simulink model "Lidar_Final_Model"  (R2022b)
settings: Solver=VariableStepAuto  StartTime=0.0  StopTime=inf  RelTol=1e-3
model workspace (MAT data in the model file):
  SL_ROS_VariableLengthArrays_MaxSizes.CommonInfo.ArrayTruncateAction = 'EmitWarning'
  SL_ROS_VariableLengthArrays_MaxSizes.MsgTypeMap = containers.Map
  SL_ROS_VariableLengthArrays_MaxSizes.MsgTypeMap.serialization.keys = {'sensor_msgs/PointCloud2', 'sensor_msgs/PointField', 'std_msgs/Header'}
  SL_ROS_VariableLengthArrays_MaxSizes.MsgTypeMap.serialization.values{1}(1).PropertyName = 'Data'
  SL_ROS_VariableLengthArrays_MaxSizes.MsgTypeMap.serialization.values{1}(1).DataType = 'uint8'
  SL_ROS_VariableLengthArrays_MaxSizes.MsgTypeMap.serialization.values{1}(1).MaxLength = 1000000
  SL_ROS_VariableLengthArrays_MaxSizes.MsgTypeMap.serialization.values{1}(2).PropertyName = 'Fields'
  SL_ROS_VariableLengthArrays_MaxSizes.MsgTypeMap.serialization.values{1}(2).DataType = 'sensor_msgs/PointField'
  SL_ROS_VariableLengthArrays_MaxSizes.MsgTypeMap.serialization.values{1}(2).MaxLength = 16
  SL_ROS_VariableLengthArrays_MaxSizes.MsgTypeMap.serialization.values{2}.PropertyName = 'Name'
  SL_ROS_VariableLengthArrays_MaxSizes.MsgTypeMap.serialization.values{2}.DataType = 'uint8'
  SL_ROS_VariableLengthArrays_MaxSizes.MsgTypeMap.serialization.values{2}.MaxLength = 200
  SL_ROS_VariableLengthArrays_MaxSizes.MsgTypeMap.serialization.values{3}.PropertyName = 'FrameId'
  SL_ROS_VariableLengthArrays_MaxSizes.MsgTypeMap.serialization.values{3}.DataType = 'uint8'
  SL_ROS_VariableLengthArrays_MaxSizes.MsgTypeMap.serialization.values{3}.MaxLength = 128
  SL_ROS_VariableLengthArrays_MaxSizes.MsgTypeMap.serialization.uniformity = 0
  SL_ROS_VariableLengthArrays_MaxSizes.MsgTypeMap.serialization.keyType = 'char'
  SL_ROS_VariableLengthArrays_MaxSizes.MsgTypeMap.serialization.valueType = 'any'
libraries: robotlib x5
settings Model: Creator=lidar  LastModifiedBy=lidar
settings OptimizationCC: EnhancedBackFolding=on  PassReuseOutputArgsAs=Individual arguments  ZeroExternalMemoryAtStartup=off  ZeroInternalMemoryAtStartup=off  MaxStackSize=64  OptimizeBlockOrder=speed  DifferentSizesBufferReuse=on  OptimizationCustomize=off  EfficientTunableParamExpr=on
settings DebuggingCC: ParameterTunabilityLossMsg=error
settings HardwareCC: ProdBitPerLong=64  ProdHWDeviceType=Intel->x86-64 (Linux 64)  UseEmbeddedCoderFeatures=off
settings RTWCC: Description=Embedded Coder  SystemTargetFile=ert.tlc  HardwareBoard=Robot Operating System (ROS)  TLCOptions="-aInlineSetEventsForThisBaseRateFcn=TLC_FALSE -aSuppressMultiTaskScheduler=TLC_FALSE  -aRateBasedStepFcn=0"  TemplateMakefile=ert_default_tmf  Toolchain=Catkin  TargetLang=C++
settings CodeAppCC: ForceParamTrailComments=on  IgnoreCustomStorageClasses=off  OperatorAnnotations=on  SimulinkDataObjDesc=on  SFDataObjDesc=on  InsertBlockDesc=on
settings ERTTargetCC: SupportNonInlinedSFcns=on

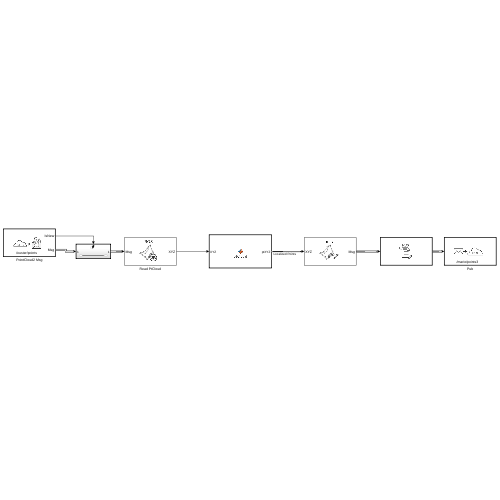
[thumbnail: Simulink's stored preview of the top-level diagram]
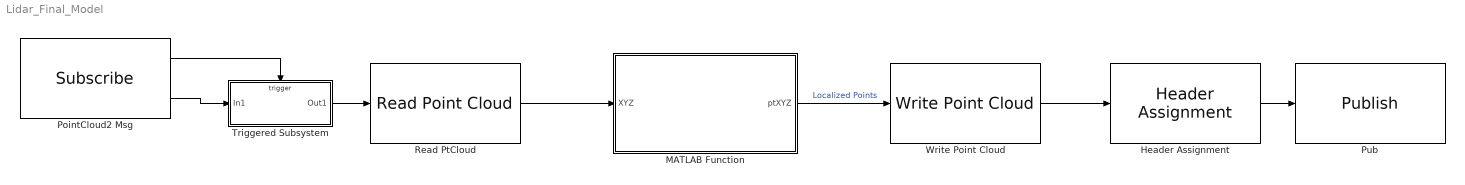
== system Lidar_Final_Model ==
  Header Assignment : robotlib/Header Assignment  SetFrameID=off  InsertTimeStamp=off  SetHeaderFieldName=Use the default Header field name  HeaderFieldName=Header
      settings: LibrarySourceBlock=roslib/ROS/Header Assignment
  MATLAB Function : MATLAB Function  TreatAsAtomicUnit=on
  PointCloud2 Msg : robotlib/Subscribe  topicSource=Select from ROS network  topic=/ouster/points  messageType=sensor_msgs/PointCloud2  SampleTime=-1  legacyBusStruct=off  messageQueueLength=1
      settings: LibrarySourceBlock=roslib/ROS/Subscribe
  Pub : robotlib/Publish  topicSource=Specify your own  topic=/mario/points3  messageType=sensor_msgs/PointCloud2  legacyBusStruct=off  messageQueueLength=1
      settings: LibrarySourceBlock=roslib/ROS/Publish
  Read PtCloud : robotlib/Read Point Cloud  MaximumPointCloudSize=[ 480, 640 ]  PreserveStructure=on  ShowRGBOutput=off  ShowIntensityOutput=off  ShowErrorCodeOutput=off  VariableSizeOutputs=off
      settings: LibrarySourceBlock=roslib/ROS/Read Point Cloud
  Triggered Subsystem : Subsystem  TreatAsAtomicUnit=on
  Write Point Cloud : robotlib/Write Point Cloud  Encoding=none  HasRGB=false  HasAlpha=false  FieldNamesStruct=struct('x', 'single', 'y', 'single', 'z', 'single')  messageType=sensor_msgs/PointCloud2
      settings: LibrarySourceBlock=roslib/ROS/Write Point Cloud
  wires:
  Read PtCloud/1 -> MATLAB Function/1(XYZ)
  MATLAB Function/1(ptXYZ) -> Write Point Cloud/1  "Localized Points"
  Header Assignment/1 -> Pub/1
  Write Point Cloud/1 -> Header Assignment/1
  Triggered Subsystem/1(Out1) -> Read PtCloud/1
  PointCloud2 Msg/2 -> Triggered Subsystem/1(In1)
  PointCloud2 Msg/1 -> Triggered Subsystem/Trigger

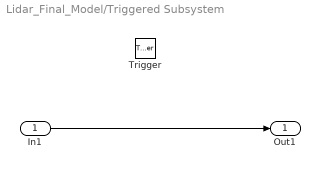
== system Lidar_Final_Model/Triggered Subsystem ==
  In1 : Inport
  Trigger : TriggerPort  VariantControl=(inherit)
  Out1 : Outport
  wires:
  In1/1 -> Out1/1

== matlab function Lidar_Final_Model/MATLAB Function ==
  data: XYZ input; ptXYZ output size=[90000 3]
%want the XYZ from the Read Point Cloud Block

function ptXYZ  = ptCloud(XYZ)

%gridStep = 0.1;


%while(1)
%ptCloud = read(obj)
%for segmenting ground - currently disabled
% groundPtsIdx = segmentGroundFromLidarData(ptCloud);
% groundPtCloud = select(ptCloud,~groundPtsIdx);

ptCloud = pointCloud(XYZ);

%downsampling - will try to publish as a test
ptCloudOut = pcdownsample(ptCloud,"random",0.15);

%reshaping the MxNx3 format point cloud into Px3 to better extract
%the XYZ coords and can be used in the Write Point Cloud Block


ptXYZ = reshape(ptCloudOut.Location, [],3);


%
%end

end
